simulink model "simulink_model"  (R2022a)
settings: Solver=VariableStepAuto  StartTime=0.0  StopTime=10.0  RelTol=1e-3
settings Model: Creator=ahmed  LastModifiedBy=ahmed

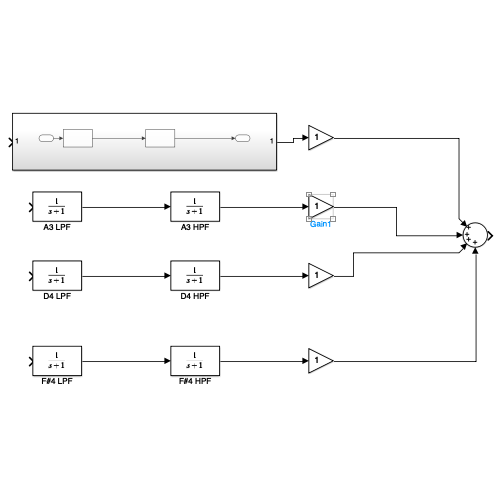
[thumbnail: Simulink's stored preview of the top-level diagram]
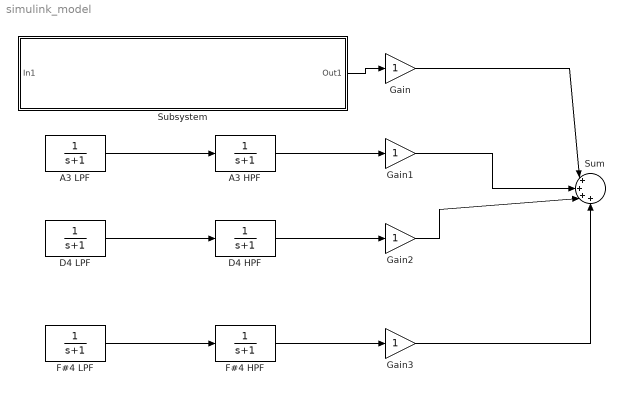
== system simulink_model ==
  A3 HPF : TransferFcn  Denominator=[1 1]
  A3 LPF : TransferFcn  Denominator=[1 1]
  D4 HPF : TransferFcn  Denominator=[1 1]
  D4 LPF : TransferFcn  Denominator=[1 1]
  F#4 HPF : TransferFcn  Denominator=[1 1]
  F#4 LPF : TransferFcn  Denominator=[1 1]
  Gain{,1..3} (4 alike) : Gain
  Subsystem : Subsystem
  Sum : Sum  Inputs=|++++
  wires:
  F#4 LPF/1 -> F#4 HPF/1
  D4 LPF/1 -> D4 HPF/1
  A3 LPF/1 -> A3 HPF/1
  F#4 HPF/1 -> Gain3/1
  D4 HPF/1 -> Gain2/1
  A3 HPF/1 -> Gain1/1
  Gain/1 -> Sum/1
  Gain1/1 -> Sum/2
  Gain2/1 -> Sum/3
  Gain3/1 -> Sum/4
  Subsystem/1(Out1) -> Gain/1

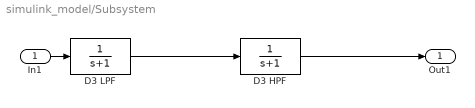
== system simulink_model/Subsystem ==
  In1 : Inport
  D3 HPF : TransferFcn  Denominator=[1 1]
  D3 LPF : TransferFcn  Denominator=[1 1]
  Out1 : Outport
  wires:
  In1/1 -> D3 LPF/1
  D3 HPF/1 -> Out1/1
  D3 LPF/1 -> D3 HPF/1
